simulink subsystem "Sensor_disturbances"  (R2021b)
settings: Solver=VariableStepAuto  StartTime=0.0  StopTime=10.0  RelTol=1e-3
undefined symbols (not defined in the file): Custom, DVL, IMU, Laser, Magnetometer, Pressure, SBL, Sonar
settings Model: Creator=esben  LastModifiedBy=esben
settings SolverCC: AlgebraicLoopSolver=TrustRegion

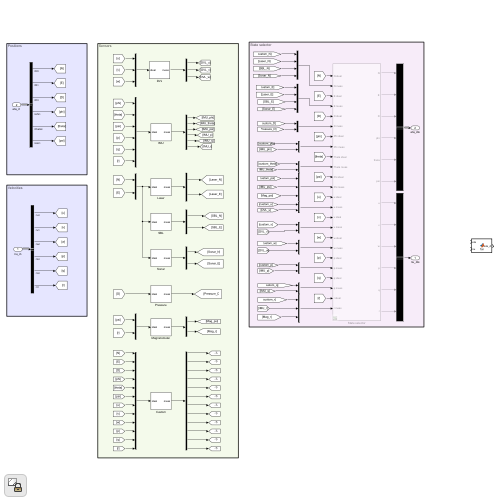
[thumbnail: Simulink's stored preview of the top-level diagram]
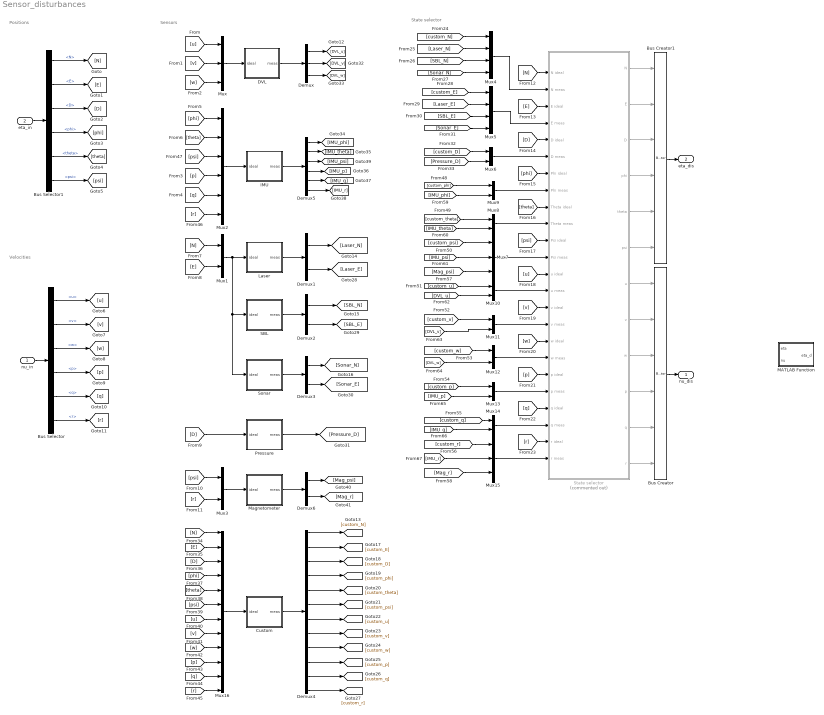
== system Sensor_disturbances ==
  note: Sensors
  note: State selector
  note: Velocities
  note: Positions
  nu_in : Inport
  eta_in : Inport  Port=2
  Bus Creator : BusCreator  Inputs=6  OutDataTypeStr=Bus: nu
      settings: InheritFromInputs=off
  Bus Creator1 : BusCreator  Inputs=6  OutDataTypeStr=Bus: eta
      settings: InheritFromInputs=off
  Bus Selector : BusSelector  OutputSignals=u,v,w,p,q,r
  Bus Selector1 : BusSelector  OutputSignals=N,E,D,phi,theta,psi
  Custom : Subsystem
  DVL : Subsystem
  Demux : Demux  Outputs=3
  Demux{1..3,6} (4 alike) : Demux  Outputs=2
  Demux4 : Demux  Outputs=12
  Demux5 : Demux  Outputs=6
  IMU : Subsystem
  Laser : Subsystem
  MATLAB Function : MATLAB Function  TreatAsAtomicUnit=on
  Magnetometer : Subsystem
  Mux : Mux  Inputs=3
  Mux{1,3,6,8..14} (10 alike) : Mux  Inputs=2
  Mux15 : Mux  Inputs=3
  Mux16 : Mux  Inputs=12
  Mux2 : Mux  Inputs=6
  Mux4 : Mux
  Mux5 : Mux
  Mux7 : Mux  Inputs=3
  Pressure : Subsystem
  SBL : Subsystem
  Sonar : Subsystem
  State selector : Subsystem  Commented=on
  nu_dis : Outport
  eta_dis : Outport  Port=2
  wires:
  eta_in/1 -> Bus Selector1/1
  nu_in/1 -> Bus Selector/1
  Sonar/1(meas) -> Demux3/1
  SBL/1(meas) -> Demux2/1
  Laser/1(meas) -> Demux1/1
  Mux1/1 -> Laser/1(ideal), SBL/1(ideal), Sonar/1(ideal)
  Bus Selector1/1 -> [N]  "<N>"
  Bus Selector1/2 -> [E]  "<E>"
  Bus Selector1/3 -> [D]  "<D>"
  Bus Selector1/4 -> [phi]  "<phi>"
  Bus Selector1/5 -> [theta]  "<theta>"
  Bus Selector1/6 -> [psi]  "<psi>"
  Bus Selector/4 -> [p]  "<p>"
  Bus Selector/1 -> [u]  "<u>"
  Bus Selector/6 -> [r]  "<r>"
  Bus Selector/2 -> [v]  "<v>"
  Bus Selector/3 -> [w]  "<w>"
  Bus Selector/5 -> [q]  "<q>"
  Mux/1 -> DVL/1(ideal)
  [u] -> Mux/1
  [v] -> Mux/2
  [w] -> Mux/3
  Mux2/1 -> IMU/1(ideal)
  [phi] -> Mux2/1
  [theta] -> Mux2/2
  [N] -> Mux1/1
  [E] -> Mux1/2
  [D] -> Pressure/1(ideal)
  Mux3/1 -> Magnetometer/1(ideal)
  [psi] -> Mux3/1
  [r] -> Mux3/2
  DVL/1(meas) -> Demux/1
  IMU/1(meas) -> Demux5/1
  Pressure/1(meas) -> [Pressure_D]
  Magnetometer/1(meas) -> Demux6/1
  Bus Creator/1 -> nu_dis/1
  Bus Creator1/1 -> eta_dis/1
  Demux/1 -> [DVL_u]
  Demux1/1 -> [Laser_N]
  Demux2/1 -> [SBL_N]
  Demux3/1 -> [Sonar_N]
  Demux4/1 -> [custom_N]
  Demux4/2 -> [custom_E]
  Demux4/6 -> [custom_psi]
  Demux4/9 -> [custom_w]
  Demux4/12 -> [custom_r]
  Demux4/11 -> [custom_q]
  Demux4/10 -> [custom_p]
  Demux4/8 -> [custom_v]
  Demux4/7 -> [custom_u]
  Demux4/5 -> [custom_theta]
  Demux4/4 -> [custom_phi]
  Demux4/3 -> [custom_D]
  Demux1/2 -> [Laser_E]
  Demux2/2 -> [SBL_E]
  Demux3/2 -> [Sonar_E]
  Demux/3 -> [DVL_w]
  Demux/2 -> [DVL_v]
  Demux5/1 -> [IMU_phi]
  Demux5/2 -> [IMU_theta]
  Demux5/3 -> [IMU_psi]
  Demux5/4 -> [IMU_p]
  Demux5/6 -> [IMU_r]
  Demux5/5 -> [IMU_q]
  Demux6/1 -> [Mag_psi]
  Demux6/2 -> [Mag_r]
  Custom/1(meas) -> Demux4/1
  Mux16/1 -> Custom/1(ideal)
  State selector/1(N) -> Bus Creator1/1
  State selector/2(E) -> Bus Creator1/2
  State selector/3(D) -> Bus Creator1/3
  State selector/4(phi) -> Bus Creator1/4
  State selector/5(theta) -> Bus Creator1/5
  State selector/6(psi) -> Bus Creator1/6
  State selector/7(u) -> Bus Creator/1
  State selector/8(v) -> Bus Creator/2
  State selector/9(w) -> Bus Creator/3
  State selector/10(p) -> Bus Creator/4
  State selector/11(q) -> Bus Creator/5
  State selector/12(r) -> Bus Creator/6
  [N] -> State selector/1(N ideal)
  [E] -> State selector/3(E ideal)
  [D] -> State selector/5(D ideal)
  [phi] -> State selector/7(Phi ideal)
  [theta] -> State selector/9(Theta ideal)
  [psi] -> State selector/11(Psi ideal)
  [u] -> State selector/13(u ideal)
  [v] -> State selector/15(v ideal)
  [w] -> State selector/17(w ideal)
  [p] -> State selector/19(p ideal)
  [q] -> State selector/21(q ideal)
  [r] -> State selector/23(r ideal)
  Mux4/1 -> State selector/2(N meas)
  [custom_N] -> Mux4/1
  [Laser_N] -> Mux4/2
  [SBL_N] -> Mux4/3
  [Sonar_N] -> Mux4/4
  Mux5/1 -> State selector/4(E meas)
  [SBL_E] -> Mux5/3
  [Laser_E] -> Mux5/2
  [custom_E] -> Mux5/1
  [Sonar_E] -> Mux5/4
  Mux6/1 -> State selector/6(D meas)
  [custom_D] -> Mux6/1
  [Pressure_D] -> Mux6/2
  [N] -> Mux16/1
  [E] -> Mux16/2
  [D] -> Mux16/3
  [phi] -> Mux16/4
  [theta] -> Mux16/5
  [psi] -> Mux16/6
  [u] -> Mux16/7
  [v] -> Mux16/8
  [w] -> Mux16/9
  [p] -> Mux16/10
  [q] -> Mux16/11
  [r] -> Mux16/12
  [q] -> Mux2/5
  [p] -> Mux2/4
  [r] -> Mux2/6
  [psi] -> Mux2/3
  Mux9/1 -> State selector/8(Phi meas)
  Mux8/1 -> State selector/10(Theta meas)
  Mux7/1 -> State selector/12(Psi meas)
  Mux10/1 -> State selector/14(u meas)
  Mux11/1 -> State selector/16(v meas)
  Mux12/1 -> State selector/18(w meas)
  Mux13/1 -> State selector/20(p meas)
  Mux14/1 -> State selector/22(q meas)
  Mux15/1 -> State selector/24(r meas)
  [custom_phi] -> Mux9/1
  [custom_theta] -> Mux8/1
  [custom_psi] -> Mux7/1
  [custom_u] -> Mux10/1
  [custom_v] -> Mux11/1
  [custom_w] -> Mux12/1
  [custom_p] -> Mux13/1
  [custom_q] -> Mux14/1
  [custom_r] -> Mux15/1
  [Mag_psi] -> Mux7/3
  [Mag_r] -> Mux15/3
  [IMU_phi] -> Mux9/2
  [IMU_theta] -> Mux8/2
  [IMU_psi] -> Mux7/2
  [DVL_u] -> Mux10/2
  [DVL_v] -> Mux11/2
  [DVL_w] -> Mux12/2
  [IMU_p] -> Mux13/2
  [IMU_q] -> Mux14/2
  [IMU_r] -> Mux15/2

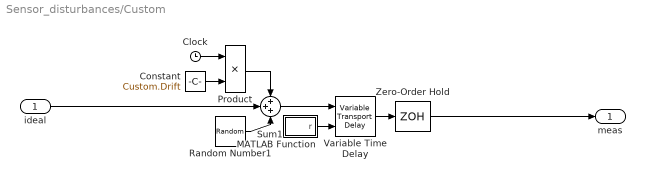
== system Sensor_disturbances/Custom ==
  ideal : Inport
  Clock : Clock
  Constant : Constant  Value=Custom.Drift
  MATLAB Function : MATLAB Function  TreatAsAtomicUnit=on  mask(Random Number (Interval)){t_min=Custom.Delay, t_max=Custom.Delay}
      mask prompts: t_min "Min Time Delay"; t_max "Max Time Delay"
      mask help: Variable Random Number between to numbers.
  Product : Product
  Random Number1 : RandomNumber  Variance=Custom.Variance  SampleTime=1/Custom.ts
  Sum1 : Sum  Inputs=+++
  Variable Time Delay : VariableTransportDelay  MaximumDelay=1000  MaximumPoints=500000  ZeroDelay=on
  Zero-Order Hold : ZeroOrderHold  SampleTime=1/Custom.ts
  meas : Outport
  wires:
  Product/1 -> Sum1/1
  Zero-Order Hold/1 -> meas/1
  Clock/1 -> Product/1
  Sum1/1 -> Variable Time Delay/1
  ideal/1 -> Sum1/2
  Constant/1 -> Product/2
  Random Number1/1 -> Sum1/3
  Variable Time Delay/1 -> Zero-Order Hold/1
  MATLAB Function/1(r) -> Variable Time Delay/2

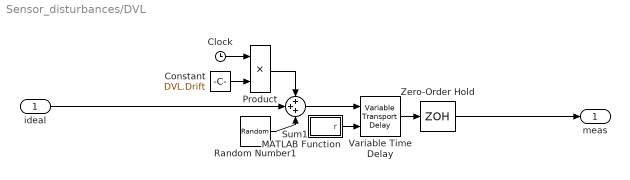
== system Sensor_disturbances/DVL ==
  ideal : Inport
  Clock : Clock
  Constant : Constant  Value=DVL.Drift
  MATLAB Function : MATLAB Function  TreatAsAtomicUnit=on  mask(Random Number (Interval)){t_min=DVL.Delay, t_max=DVL.Delay}
      mask prompts: t_min "Min Time Delay"; t_max "Max Time Delay"
      mask help: Variable Random Number between to numbers.
  Product : Product
  Random Number1 : RandomNumber  Variance=DVL.Variance  SampleTime=1/DVL.ts
  Sum1 : Sum  Inputs=+++
  Variable Time Delay : VariableTransportDelay  MaximumDelay=1000  MaximumPoints=500000  ZeroDelay=on
  Zero-Order Hold : ZeroOrderHold  SampleTime=1/DVL.ts
  meas : Outport
  wires:
  Zero-Order Hold/1 -> meas/1
  ideal/1 -> Sum1/2
  Product/1 -> Sum1/1
  Clock/1 -> Product/1
  Sum1/1 -> Variable Time Delay/1
  Constant/1 -> Product/2
  Random Number1/1 -> Sum1/3
  Variable Time Delay/1 -> Zero-Order Hold/1
  MATLAB Function/1(r) -> Variable Time Delay/2

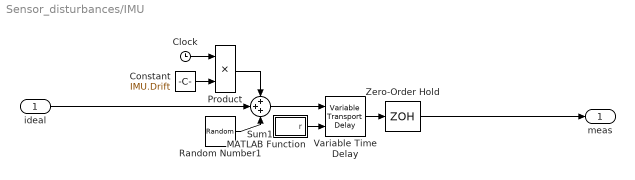
== system Sensor_disturbances/IMU ==
  ideal : Inport
  Clock : Clock
  Constant : Constant  Value=IMU.Drift
  MATLAB Function : MATLAB Function  TreatAsAtomicUnit=on  mask(Random Number (Interval)){t_min=IMU.Delay, t_max=IMU.Delay}
      mask prompts: t_min "Min Time Delay"; t_max "Max Time Delay"
      mask help: Variable Random Number between to numbers.
  Product : Product
  Random Number1 : RandomNumber  Variance=IMU.Variance  SampleTime=1/IMU.ts
  Sum1 : Sum  Inputs=+++
  Variable Time Delay : VariableTransportDelay  MaximumDelay=1000  MaximumPoints=500000  ZeroDelay=on
  Zero-Order Hold : ZeroOrderHold  SampleTime=1/IMU.ts
  meas : Outport
  wires:
  MATLAB Function/1(r) -> Variable Time Delay/2
  Variable Time Delay/1 -> Zero-Order Hold/1
  Random Number1/1 -> Sum1/3
  Constant/1 -> Product/2
  ideal/1 -> Sum1/2
  Sum1/1 -> Variable Time Delay/1
  Clock/1 -> Product/1
  Zero-Order Hold/1 -> meas/1
  Product/1 -> Sum1/1

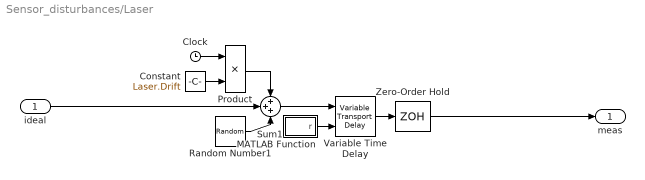
== system Sensor_disturbances/Laser ==
  ideal : Inport
  Clock : Clock
  Constant : Constant  Value=Laser.Drift
  MATLAB Function : MATLAB Function  TreatAsAtomicUnit=on  mask(Random Number (Interval)){t_min=Laser.Delay, t_max=Laser.Delay}
      mask prompts: t_min "Min Time Delay"; t_max "Max Time Delay"
      mask help: Variable Random Number between to numbers.
  Product : Product
  Random Number1 : RandomNumber  Variance=Laser.Variance  SampleTime=1/Laser.ts
  Sum1 : Sum  Inputs=+++
  Variable Time Delay : VariableTransportDelay  MaximumDelay=1000  MaximumPoints=500000  ZeroDelay=on
  Zero-Order Hold : ZeroOrderHold  SampleTime=1/Laser.ts
  meas : Outport
  wires:
  Product/1 -> Sum1/1
  Zero-Order Hold/1 -> meas/1
  Clock/1 -> Product/1
  Sum1/1 -> Variable Time Delay/1
  ideal/1 -> Sum1/2
  Constant/1 -> Product/2
  Random Number1/1 -> Sum1/3
  Variable Time Delay/1 -> Zero-Order Hold/1
  MATLAB Function/1(r) -> Variable Time Delay/2

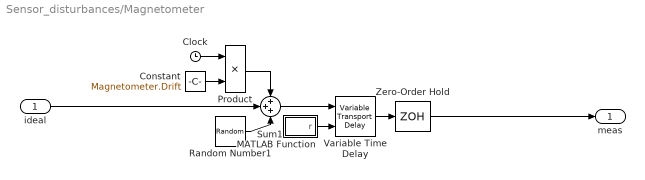
== system Sensor_disturbances/Magnetometer ==
  ideal : Inport
  Clock : Clock
  Constant : Constant  Value=Magnetometer.Drift
  MATLAB Function : MATLAB Function  TreatAsAtomicUnit=on  mask(Random Number (Interval)){t_min=Magnetometer.Delay, t_max=Magnetometer.Delay}
      mask prompts: t_min "Min Time Delay"; t_max "Max Time Delay"
      mask help: Variable Random Number between to numbers.
  Product : Product
  Random Number1 : RandomNumber  Variance=Magnetometer.Variance  SampleTime=1/Magnetometer.ts
  Sum1 : Sum  Inputs=+++
  Variable Time Delay : VariableTransportDelay  MaximumDelay=1000  MaximumPoints=500000  ZeroDelay=on
  Zero-Order Hold : ZeroOrderHold  SampleTime=1/Magnetometer.ts
  meas : Outport
  wires:
  MATLAB Function/1(r) -> Variable Time Delay/2
  Variable Time Delay/1 -> Zero-Order Hold/1
  Random Number1/1 -> Sum1/3
  Constant/1 -> Product/2
  ideal/1 -> Sum1/2
  Sum1/1 -> Variable Time Delay/1
  Clock/1 -> Product/1
  Zero-Order Hold/1 -> meas/1
  Product/1 -> Sum1/1

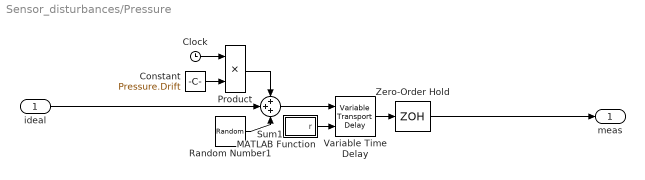
== system Sensor_disturbances/Pressure ==
  ideal : Inport
  Clock : Clock
  Constant : Constant  Value=Pressure.Drift
  MATLAB Function : MATLAB Function  TreatAsAtomicUnit=on  mask(Random Number (Interval)){t_min=Pressure.Delay, t_max=Pressure.Delay}
      mask prompts: t_min "Min Time Delay"; t_max "Max Time Delay"
      mask help: Variable Random Number between to numbers.
  Product : Product
  Random Number1 : RandomNumber  Variance=Pressure.Variance  SampleTime=1/Pressure.ts
  Sum1 : Sum  Inputs=+++
  Variable Time Delay : VariableTransportDelay  MaximumDelay=1000  MaximumPoints=500000  ZeroDelay=on
  Zero-Order Hold : ZeroOrderHold  SampleTime=1/Pressure.ts
  meas : Outport
  wires:
  Product/1 -> Sum1/1
  Zero-Order Hold/1 -> meas/1
  Clock/1 -> Product/1
  Sum1/1 -> Variable Time Delay/1
  ideal/1 -> Sum1/2
  Constant/1 -> Product/2
  Random Number1/1 -> Sum1/3
  Variable Time Delay/1 -> Zero-Order Hold/1
  MATLAB Function/1(r) -> Variable Time Delay/2

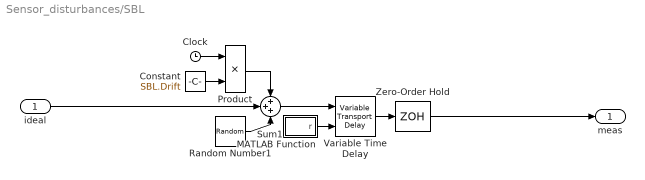
== system Sensor_disturbances/SBL ==
  ideal : Inport
  Clock : Clock
  Constant : Constant  Value=SBL.Drift
  MATLAB Function : MATLAB Function  TreatAsAtomicUnit=on  mask(Random Number (Interval)){t_min=SBL.Delay, t_max=SBL.Delay}
      mask prompts: t_min "Min Time Delay"; t_max "Max Time Delay"
      mask help: Variable Random Number between to numbers.
  Product : Product
  Random Number1 : RandomNumber  Variance=SBL.Variance  SampleTime=1/SBL.ts
  Sum1 : Sum  Inputs=+++
  Variable Time Delay : VariableTransportDelay  MaximumDelay=1000  MaximumPoints=500000  ZeroDelay=on
  Zero-Order Hold : ZeroOrderHold  SampleTime=1/SBL.ts
  meas : Outport
  wires:
  MATLAB Function/1(r) -> Variable Time Delay/2
  Variable Time Delay/1 -> Zero-Order Hold/1
  Random Number1/1 -> Sum1/3
  Constant/1 -> Product/2
  ideal/1 -> Sum1/2
  Sum1/1 -> Variable Time Delay/1
  Clock/1 -> Product/1
  Zero-Order Hold/1 -> meas/1
  Product/1 -> Sum1/1

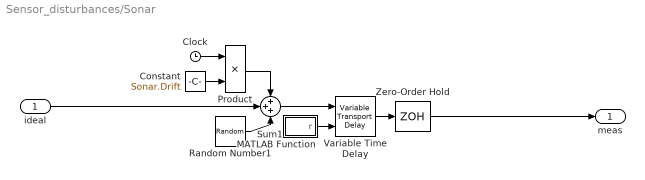
== system Sensor_disturbances/Sonar ==
  ideal : Inport
  Clock : Clock
  Constant : Constant  Value=Sonar.Drift
  MATLAB Function : MATLAB Function  TreatAsAtomicUnit=on  mask(Random Number (Interval)){t_min=Sonar.Delay, t_max=Sonar.Delay}
      mask prompts: t_min "Min Time Delay"; t_max "Max Time Delay"
      mask help: Variable Random Number between to numbers.
  Product : Product
  Random Number1 : RandomNumber  Variance=Sonar.Variance  SampleTime=1/Sonar.ts
  Sum1 : Sum  Inputs=+++
  Variable Time Delay : VariableTransportDelay  MaximumDelay=1000  MaximumPoints=500000  ZeroDelay=on
  Zero-Order Hold : ZeroOrderHold  SampleTime=1/Sonar.ts
  meas : Outport
  wires:
  Product/1 -> Sum1/1
  Zero-Order Hold/1 -> meas/1
  Clock/1 -> Product/1
  Sum1/1 -> Variable Time Delay/1
  ideal/1 -> Sum1/2
  Constant/1 -> Product/2
  Random Number1/1 -> Sum1/3
  Variable Time Delay/1 -> Zero-Order Hold/1
  MATLAB Function/1(r) -> Variable Time Delay/2

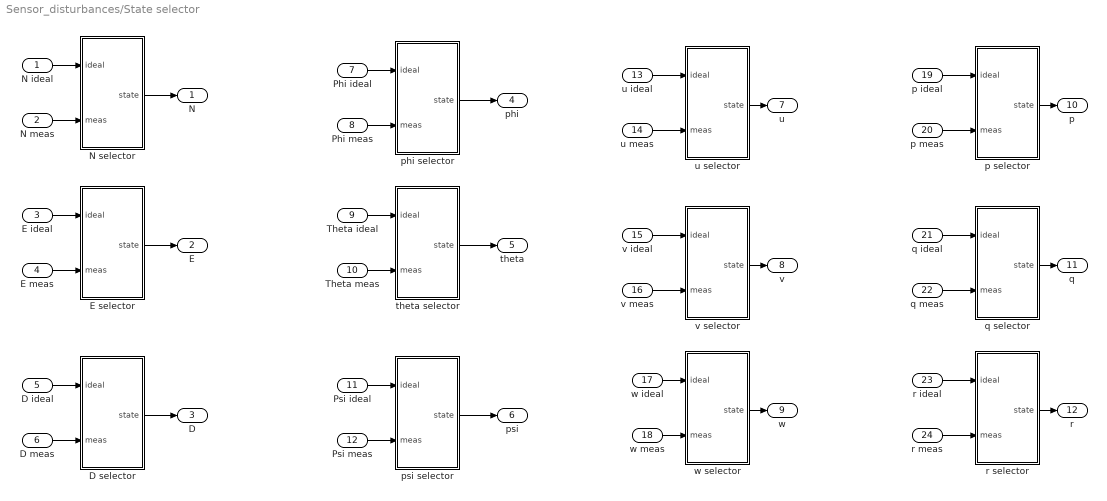
== system Sensor_disturbances/State selector ==
  N ideal : Inport
  N meas : Inport  Port=2
  E ideal : Inport  Port=3
  E meas : Inport  Port=4
  D ideal : Inport  Port=5
  D meas : Inport  Port=6
  Phi ideal : Inport  Port=7
  Phi meas : Inport  Port=8
  Theta ideal : Inport  Port=9
  Theta meas : Inport  Port=10
  Psi ideal : Inport  Port=11
  Psi meas : Inport  Port=12
  u ideal : Inport  Port=13
  u meas : Inport  Port=14
  v ideal : Inport  Port=15
  v meas : Inport  Port=16
  w ideal : Inport  Port=17
  w meas : Inport  Port=18
  p ideal : Inport  Port=19
  p meas : Inport  Port=20
  q ideal : Inport  Port=21
  q meas : Inport  Port=22
  r ideal : Inport  Port=23
  r meas : Inport  Port=24
  D selector : MATLAB Function  TreatAsAtomicUnit=on
  E selector : MATLAB Function  TreatAsAtomicUnit=on
  N selector : MATLAB Function  TreatAsAtomicUnit=on
  p selector : MATLAB Function  TreatAsAtomicUnit=on
  phi selector : MATLAB Function  TreatAsAtomicUnit=on
  psi selector : MATLAB Function  TreatAsAtomicUnit=on
  q selector : MATLAB Function  TreatAsAtomicUnit=on
  r selector : MATLAB Function  TreatAsAtomicUnit=on
  theta selector : MATLAB Function  TreatAsAtomicUnit=on
  u selector : MATLAB Function  TreatAsAtomicUnit=on
  v selector : MATLAB Function  TreatAsAtomicUnit=on
  w selector : MATLAB Function  TreatAsAtomicUnit=on
  N : Outport
  E : Outport  Port=2
  D : Outport  Port=3
  phi : Outport  Port=4
  theta : Outport  Port=5
  psi : Outport  Port=6
  u : Outport  Port=7
  v : Outport  Port=8
  w : Outport  Port=9
  p : Outport  Port=10
  q : Outport  Port=11
  r : Outport  Port=12
  wires:
  q meas/1 -> q selector/2(meas)
  p meas/1 -> p selector/2(meas)
  w meas/1 -> w selector/2(meas)
  v meas/1 -> v selector/2(meas)
  u meas/1 -> u selector/2(meas)
  Theta meas/1 -> theta selector/2(meas)
  Phi meas/1 -> phi selector/2(meas)
  D meas/1 -> D selector/2(meas)
  r selector/1(state) -> r/1
  u selector/1(state) -> u/1
  Theta ideal/1 -> theta selector/1(ideal)
  N meas/1 -> N selector/2(meas)
  D selector/1(state) -> D/1
  psi selector/1(state) -> psi/1
  q ideal/1 -> q selector/1(ideal)
  q selector/1(state) -> q/1
  N ideal/1 -> N selector/1(ideal)
  p selector/1(state) -> p/1
  v selector/1(state) -> v/1
  N selector/1(state) -> N/1
  Phi ideal/1 -> phi selector/1(ideal)
  D ideal/1 -> D selector/1(ideal)
  E meas/1 -> E selector/2(meas)
  v ideal/1 -> v selector/1(ideal)
  p ideal/1 -> p selector/1(ideal)
  r ideal/1 -> r selector/1(ideal)
  w ideal/1 -> w selector/1(ideal)
  u ideal/1 -> u selector/1(ideal)
  theta selector/1(state) -> theta/1
  w selector/1(state) -> w/1
  Psi meas/1 -> psi selector/2(meas)
  r meas/1 -> r selector/2(meas)
  Psi ideal/1 -> psi selector/1(ideal)
  E selector/1(state) -> E/1
  E ideal/1 -> E selector/1(ideal)
  phi selector/1(state) -> phi/1

== matlab function Sensor_disturbances/State selector/phi selector ==
  data: ideal input; meas input; state output; Sim_param parameter
function state = fcn(ideal,meas,Sim_param)
    sen_sel = Sim_param.States.phi;
        
    switch sen_sel
        case 8
            state = meas(1); % custom sensor
        case 2
            state = meas(2); % pressure
        otherwise
            state = ideal;
    end

== matlab function Sensor_disturbances/Laser/MATLAB Function ==
  data: r output; t_min parameter; t_max parameter
function r = fcn(t_min, t_max)

r = (t_max-t_min).*rand(1,1) + t_min;

== matlab function Sensor_disturbances/State selector/theta selector ==
  data: ideal input; meas input; state output; Sim_param parameter
function state = fcn(ideal,meas,Sim_param)
    sen_sel = Sim_param.States.theta;
        
    switch sen_sel
        case 8
            state = meas(1); % custom sensor
        case 2
            state = meas(2); % pressure
        otherwise
            state = ideal;
    end

== matlab function Sensor_disturbances/State selector/u selector ==
  data: ideal input; meas input; state output; Sim_param parameter
function state = fcn(ideal,meas,Sim_param)
    sen_sel = Sim_param.States.u;
        
    switch sen_sel
        case 8
            state = meas(1); % custom sensor
        case 1
            state = meas(2); % pressure
        otherwise
            state = ideal;
    end

== matlab function Sensor_disturbances/State selector/v selector ==
  data: ideal input; meas input; state output; Sim_param parameter
function state = fcn(ideal,meas,Sim_param)
    sen_sel = Sim_param.States.v;
        
    switch sen_sel
        case 8
            state = meas(1); % custom sensor
        case 1
            state = meas(2); % pressure
        otherwise
            state = ideal;
    end

== matlab function Sensor_disturbances/State selector/w selector ==
  data: ideal input; meas input; state output; Sim_param parameter
function state = fcn(ideal,meas,Sim_param)
    sen_sel = Sim_param.States.w;
        
    switch sen_sel
        case 8
            state = meas(1); % custom sensor
        case 1
            state = meas(2); % pressure
        otherwise
            state = ideal;
    end

== matlab function Sensor_disturbances/State selector/psi selector ==
  data: ideal input; meas input; state output; Sim_param parameter
function state = fcn(ideal,meas,Sim_param)
    sen_sel = Sim_param.States.psi;
        
    switch sen_sel
        case 8
            state = meas(1); % custom sensor
        case 2
            state = meas(2); % IMU
        case 4
            state = meas(3); % Magnetometer
        otherwise
            state = ideal;
    end

== matlab function Sensor_disturbances/State selector/p selector ==
  data: ideal input; meas input; state output; Sim_param parameter
function state = fcn(ideal,meas,Sim_param)
    sen_sel = Sim_param.States.p;
        
    switch sen_sel
        case 8
            state = meas(1); % custom sensor
        case 2
            state = meas(2); % pressure
        otherwise
            state = ideal;
    end

== matlab function Sensor_disturbances/State selector/q selector ==
  data: ideal input; meas input; state output; Sim_param parameter
function state = fcn(ideal,meas,Sim_param)
    sen_sel = Sim_param.States.q;
        
    switch sen_sel
        case 8
            state = meas(1); % custom sensor
        case 2
            state = meas(2); % pressure
        otherwise
            state = ideal;
    end

== matlab function Sensor_disturbances/State selector/r selector ==
  data: ideal input; meas input; state output; Sim_param parameter
function state = fcn(ideal,meas,Sim_param)
    sen_sel = Sim_param.States.r;
        
    switch sen_sel
        case 8
            state = meas(1); % custom sensor
        case 2
            state = meas(2); % pressure
        case 4
            state = meas(3); % pressure
        otherwise
            state = ideal;
    end

== matlab function Sensor_disturbances/Custom/MATLAB Function ==
  data: r output; t_min parameter; t_max parameter
function r = fcn(t_min, t_max)

r = (t_max-t_min).*rand(1,1) + t_min;

== matlab function Sensor_disturbances/Magnetometer/MATLAB Function ==
  data: r output; t_min parameter; t_max parameter
function r = fcn(t_min, t_max)

r = (t_max-t_min).*rand(1,1) + t_min;

== matlab function Sensor_disturbances/IMU/MATLAB Function ==
  data: r output; t_min parameter; t_max parameter
function r = fcn(t_min, t_max)

r = (t_max-t_min).*rand(1,1) + t_min;

== matlab function Sensor_disturbances/SBL/MATLAB Function ==
  data: r output; t_min parameter; t_max parameter
function r = fcn(t_min, t_max)

r = (t_max-t_min).*rand(1,1) + t_min;

== matlab function Sensor_disturbances/Sonar/MATLAB Function ==
  data: r output; t_min parameter; t_max parameter
function r = fcn(t_min, t_max)

r = (t_max-t_min).*rand(1,1) + t_min;

== matlab function Sensor_disturbances/Pressure/MATLAB Function ==
  data: r output; t_min parameter; t_max parameter
function r = fcn(t_min, t_max)

r = (t_max-t_min).*rand(1,1) + t_min;

== matlab function Sensor_disturbances/DVL/MATLAB Function ==
  data: r output; t_min parameter; t_max parameter
function r = fcn(t_min, t_max)

r = (t_max-t_min).*rand(1,1) + t_min;

== matlab function Sensor_disturbances/State selector/N selector ==
  data: ideal input; meas input; state output; Sim_param parameter
function state = fcn(ideal,meas,Sim_param)
    sen_sel = Sim_param.States.N;
  
    switch sen_sel
        case 8
            state = meas(1); % custom sensor
        case 3
            state = meas(2); % laser
        case 6
            state = meas(3); % SBL
        case 7
            state = meas(4); % Sonar
        otherwise
            state = ideal;
    end

== matlab function Sensor_disturbances/State selector/E selector ==
  data: ideal input; meas input; state output; Sim_param parameter
function state = fcn(ideal,meas,Sim_param)
    sen_sel = Sim_param.States.E;
        
    switch sen_sel
        case 8
            state = meas(1); % custom sensor
        case 3
            state = meas(2); % laser
        case 6
            state = meas(3); % SBL
        case 7
            state = meas(4); % Sonar
        otherwise
            state = ideal;
    end

== matlab function Sensor_disturbances/MATLAB Function ==
  data: eta input Bus: eta; nu input Bus: nu; eta_d output
function eta_d = fcn(eta,nu)

eta_d = [Rotn_b(eta.phi,eta.theta,eta.psi) zeros(3,3);zeros(3,3) TransAng(eta.phi,eta.theta,eta.psi)]*struct2vec(nu);

== matlab function Sensor_disturbances/State selector/D selector ==
  data: ideal input; meas input; state output; Sim_param parameter
function state = fcn(ideal,meas,Sim_param)
    sen_sel = Sim_param.States.D;
        
    switch sen_sel
        case 8
            state = meas(1); % custom sensor
        case 5
            state = meas(2); % pressure
        otherwise
            state = ideal;
    end
